simulink model "typicaldianlidianzi"  (R2016a)
settings: Solver=VariableStepAuto  StartTime=0.0  StopTime=150e-3  RelTol=1e-3
libraries: powerlib x19
settings Model: Creator=24535  LastModifiedBy=24535

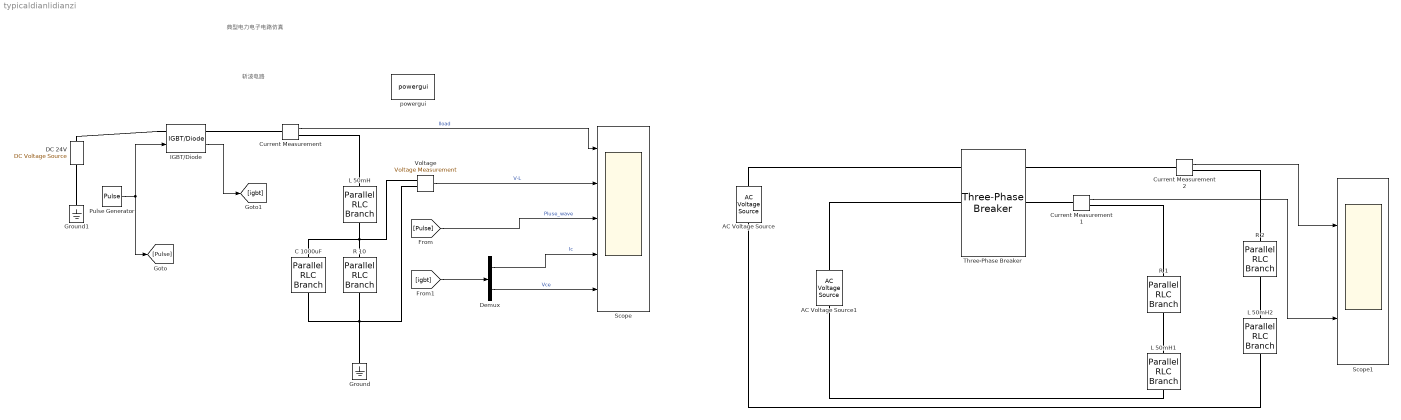
== system typicaldianlidianzi ==
  note: 斩波电路
  note: 典型电力电子电路仿真
  AC Voltage Source : powerlib/Electrical Sources/AC Voltage Source  Amplitude=5000  Phase=0  Frequency=50  SampleTime=0  Measurements=None  BusType=swing  Pref=10e3  Qref=0  Qmin=-inf  Qmax=+inf
  AC Voltage Source1 : powerlib/Electrical Sources/AC Voltage Source  Amplitude=5000  Phase=0  Frequency=50  SampleTime=0  Measurements=None  BusType=swing  Pref=10e3  Qref=0  Qmin=-inf  Qmax=+inf
  C 1000uF : powerlib/Elements/Parallel RLC Branch  LConnTagsString=a  RConnTagsString=__new0  BranchType=C  Resistance=1  Inductance=1e-3  SetiL0=off  InitialCurrent=0  Capacitance=1000e-6  Setx0=off  InitialVoltage=0  Measurements=None
  Current Measurement : powerlib/Measurements/Current Measurement  PhasorSimulation=off  OutputType=Complex  PSBequivalent=0
  Current Measurement1 : powerlib/Measurements/Current Measurement  PhasorSimulation=off  OutputType=Complex  PSBequivalent=0
  Current Measurement2 : powerlib/Measurements/Current Measurement  PhasorSimulation=off  OutputType=Complex  PSBequivalent=0
  DC 24V : powerlib/Electrical Sources/DC Voltage Source  Amplitude=24  Measurements=None
  Demux : Demux  Outputs=2
  Ground : powerlib/Elements/Ground  LConnTagsString=a
  Ground1 : powerlib/Elements/Ground  LConnTagsString=a
  IGBT/Diode : powerlib/Power Electronics/IGBT//Diode  Ron=1e-3  Rs=100  Cs=4.7e-6  Measurements=on
  L 50mH : powerlib/Elements/Parallel RLC Branch  LConnTagsString=a  RConnTagsString=__new0  BranchType=L  Resistance=1  Inductance=50e-3  SetiL0=off  InitialCurrent=0  Capacitance=1e-6  Setx0=off  InitialVoltage=0  Measurements=None
  L 50mH1 : powerlib/Elements/Parallel RLC Branch  LConnTagsString=a  RConnTagsString=__new0  BranchType=L  Resistance=1  Inductance=50e-3  SetiL0=off  InitialCurrent=0  Capacitance=1e-6  Setx0=off  InitialVoltage=0  Measurements=None
  L 50mH2 : powerlib/Elements/Parallel RLC Branch  LConnTagsString=a  RConnTagsString=__new0  BranchType=L  Resistance=1  Inductance=50e-3  SetiL0=off  InitialCurrent=0  Capacitance=1e-6  Setx0=off  InitialVoltage=0  Measurements=None
  Pulse Generator : DiscretePulseGenerator  PulseType=Time based  Period=1e-3  PulseWidth=50
  R 1 : powerlib/Elements/Parallel RLC Branch  LConnTagsString=a  RConnTagsString=__new0  BranchType=R  Resistance=10  Inductance=1e-3  SetiL0=off  InitialCurrent=0  Capacitance=1e-6  Setx0=off  InitialVoltage=0  Measurements=None
  R 10 : powerlib/Elements/Parallel RLC Branch  LConnTagsString=a  RConnTagsString=__new0  BranchType=R  Resistance=10  Inductance=1e-3  SetiL0=off  InitialCurrent=0  Capacitance=1e-6  Setx0=off  InitialVoltage=0  Measurements=None
  R 2 : powerlib/Elements/Parallel RLC Branch  LConnTagsString=a  RConnTagsString=__new0  BranchType=R  Resistance=10  Inductance=1e-3  SetiL0=off  InitialCurrent=0  Capacitance=1e-6  Setx0=off  InitialVoltage=0  Measurements=None
  Scope : Scope  NumInputPorts=5
  Scope1 : Scope  NumInputPorts=2
  Three-Phase Breaker : powerlib/Elements/Three-Phase Breaker  InitialState=closed  SwitchA=on  SwitchB=on  SwitchC=on  SwitchTimes="[0.02  0.1]"  External=off  BreakerResistance=0.01  SnubberResistance=1e6  SnubberCapacitance=inf  Measurements=None
  Voltage : powerlib/Measurements/Voltage Measurement  PhasorSimulation=off  OutputType=Complex  PSBequivalent=0
  powergui : powerlib/powergui  Priority=1  SimulationMode=Continuous  SolverType=Tustin/Backward Euler (TBE)  SampleTime=50e-6  frequency=60  SPID=off  DisableSnubberDevices=off  DisableRonSwitches=off  DisableVfSwitches=off  SwTol=0  DisplayEquations=off  Interpol=off  ExternalGateDelay=off  methode=off  Ts=10  FunctionMessages=off  echomessages=off  HookPort=off  EnableUseOfTLC=off  x0status=blocks  frequencyindice=0  Pbase=100e6  ErrMax=1e-4  Iterations=50  UnitsV=kV  UnitsW=MW  buscounter=0  RestoreLinks=warning  ResistiveCurrentMeasurement=off  Frange=[0:2:500]  Ylog=off  Xlog=on  ShowGrid=off  save=off  variable=ZData  structure=0  ZoomFFT=off  StartTime=0.0  cycles=1  DisplayStyle=1  fundamental=60  FreqAxis=off  MaxFrequency=1000  frequencyindicesteady=1  RmsSteady=1  display=off
  wires:
  [Pulse] -> Scope/3  "Pluse_wave"
  Pulse Generator/1 -> [Pulse], IGBT/Diode/1
  [igbt] -> Demux/1
  IGBT/Diode/1 -> [igbt]
  Demux/1 -> Scope/4  "Ic"
  Demux/2 -> Scope/5  "Vce"
  Current Measurement/1 -> Scope/1  "Iload"
  Voltage/1 -> Scope/2  "V-L"
  Current Measurement2/1 -> Scope1/1
  Current Measurement1/1 -> Scope1/2
  connections:
  L 50mH/LConn1 -- Current Measurement/RConn1
  L 50mH/RConn1 -- Voltage/LConn1 -- C 1000uF/LConn1 -- R 10/LConn1
  Ground/LConn1 -- R 10/RConn1 -- Voltage/LConn2 -- C 1000uF/RConn1
  Ground1/LConn1 -- DC 24V/LConn1
  IGBT/Diode/LConn1 -- DC 24V/RConn1
  IGBT/Diode/RConn1 -- Current Measurement/LConn1
  Current Measurement1/LConn1 -- Three-Phase Breaker/RConn2
  L 50mH1/LConn1 -- R 1/RConn1
  Current Measurement1/RConn1 -- R 1/LConn1
  L 50mH1/RConn1 -- AC Voltage Source1/LConn1
  AC Voltage Source1/RConn1 -- Three-Phase Breaker/LConn2
  AC Voltage Source/RConn1 -- Three-Phase Breaker/LConn1
  Current Measurement2/LConn1 -- Three-Phase Breaker/RConn1
  Current Measurement2/RConn1 -- R 2/LConn1
  L 50mH2/LConn1 -- R 2/RConn1
  L 50mH2/RConn1 -- AC Voltage Source/LConn1
